simulink library "gnc2_interface_lib"  (R2016b)
settings: Solver=VariableStepAuto  StartTime=0.0  StopTime=10.0  RelTol=1e-3
undefined symbols (not defined in the file): soac_params
libraries: simulink x2, gnc2_lib x1
settings Model: Creator=taylorreynolds  LastModifiedBy=Taylor

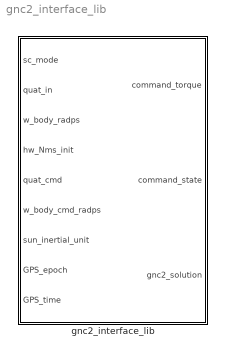
== system gnc2_interface_lib ==
  gnc2_interface_lib : Subsystem

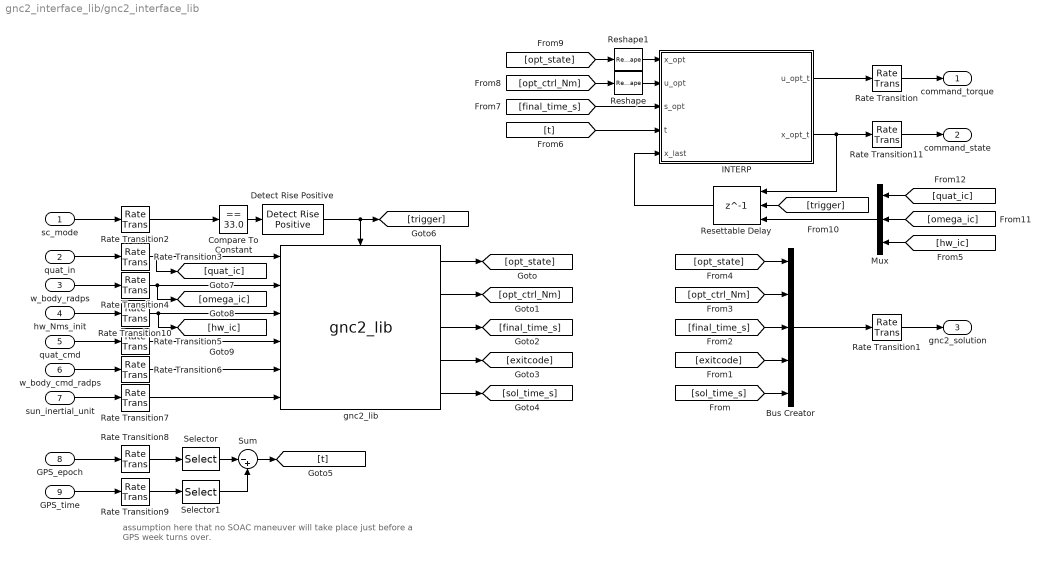
== system gnc2_interface_lib/gnc2_interface_lib ==
  note: assumption here that no SOAC maneuver will take place just
      | before a GPS week turns over.
  sc_mode : Inport
  quat_in : Inport  Port=2
  w_body_radps : Inport  Port=3
  hw_Nms_init : Inport  Port=4
  quat_cmd : Inport  Port=5
  w_body_cmd_radps : Inport  Port=6
  sun_inertial_unit : Inport  Port=7
  GPS_epoch : Inport  Port=8
  GPS_time : Inport  Port=9
  Bus Creator : BusCreator  Inputs=5
  Compare To Constant : simulink/Logic and Bit Operations/Compare To Constant  relop===  const=33.0  OutDataTypeStr=boolean
  Detect Rise Positive : simulink/Logic and Bit Operations/Detect Rise Positive  vinit=0  OutDataTypeStr=boolean
  INTERP : MATLAB Function  TreatAsAtomicUnit=on
  Mux : Mux  Inputs=[4 3 3]
  Rate Transition : RateTransition  X0=soac_params.ic.cmd_torque
  Rate Transition1 : RateTransition
  Rate Transition10 : RateTransition  X0=soac_params.ic.hw_Nms  OutPortSampleTime=soac_params.sample_time_s
  Rate Transition11 : RateTransition  X0=soac_params.ic.cmd_state
  Rate Transition2 : RateTransition  X0=soac_params.ic.sc_mode  OutPortSampleTime=soac_params.sample_time_s
  Rate Transition3 : RateTransition  X0=soac_params.ic.quat_in  OutPortSampleTime=soac_params.sample_time_s
  Rate Transition4 : RateTransition  X0=soac_params.ic.w_body_radps  OutPortSampleTime=soac_params.sample_time_s
  Rate Transition5 : RateTransition  X0=soac_params.ic.quat_cmd  OutPortSampleTime=soac_params.sample_time_s
  Rate Transition6 : RateTransition  X0=soac_params.ic.w_body_cmd_radps  OutPortSampleTime=soac_params.sample_time_s
  Rate Transition7 : RateTransition  X0=soac_params.ic.sun_inertial_unit  OutPortSampleTime=soac_params.sample_time_s
  Rate Transition8 : RateTransition  X0=soac_params.ic.gps_epoch_s  OutPortSampleTime=soac_params.sample_time_s
  Rate Transition9 : RateTransition  X0=soac_params.ic.gps_time_s  OutPortSampleTime=soac_params.sample_time_s
  Resettable Delay : Delay  DelayLength=1  InitialConditionSource=Input port  ExternalReset=Rising
      settings: InputPortMap=u0,r5,p4
  Reshape : Reshape  OutputDimensionality=Customize  OutputDimensions=[3,soac_params.N]
  Reshape1 : Reshape  OutputDimensionality=Customize  OutputDimensions=[10,soac_params.N]
  Selector : Selector  InputPortWidth=2  IndexOptions=Index vector (dialog)  Indices=1  OutputSizes=1
  Selector1 : Selector  InputPortWidth=2  IndexOptions=Index vector (dialog)  Indices=1  OutputSizes=1
  Sum : Sum  Inputs=|-+
  gnc2_lib : gnc2_lib/gnc2_lib
  command_torque : Outport
  command_state : Outport  Port=2
  gnc2_solution : Outport  Port=3
  wires:
  Reshape1/1 -> INTERP/1(x_opt)
  [t] -> INTERP/4(t)
  [final_time_s] -> INTERP/3(s_opt)
  [opt_ctrl_Nm] -> Reshape/1
  [opt_state] -> Reshape1/1
  Reshape/1 -> INTERP/2(u_opt)
  Resettable Delay/1 -> INTERP/5(x_last)
  Rate Transition11/1 -> command_state/1
  INTERP/2(x_opt_t) -> Resettable Delay/1, Rate Transition11/1
  INTERP/1(u_opt_t) -> Rate Transition/1
  quat_in/1 -> Rate Transition3/1
  w_body_radps/1 -> Rate Transition4/1
  quat_cmd/1 -> Rate Transition5/1
  w_body_cmd_radps/1 -> Rate Transition6/1
  sun_inertial_unit/1 -> Rate Transition7/1
  sc_mode/1 -> Rate Transition2/1
  Compare To Constant/1 -> Detect Rise Positive/1
  gnc2_lib/1 -> [opt_state]
  gnc2_lib/5 -> [sol_time_s]
  gnc2_lib/4 -> [exitcode]
  gnc2_lib/3 -> [final_time_s]
  gnc2_lib/2 -> [opt_ctrl_Nm]
  GPS_epoch/1 -> Rate Transition8/1
  GPS_time/1 -> Rate Transition9/1
  Sum/1 -> [t]
  Bus Creator/1 -> Rate Transition1/1
  [sol_time_s] -> Bus Creator/5
  [exitcode] -> Bus Creator/4
  [final_time_s] -> Bus Creator/3
  [opt_ctrl_Nm] -> Bus Creator/2
  [opt_state] -> Bus Creator/1
  Rate Transition/1 -> command_torque/1
  Rate Transition1/1 -> gnc2_solution/1
  Rate Transition2/1 -> Compare To Constant/1
  Rate Transition3/1 -> [quat_ic], gnc2_lib/1
  Rate Transition4/1 -> [omega_ic], gnc2_lib/2
  Rate Transition5/1 -> gnc2_lib/4
  Rate Transition6/1 -> gnc2_lib/5
  Rate Transition7/1 -> gnc2_lib/6
  Rate Transition8/1 -> Selector/1
  Rate Transition9/1 -> Selector1/1
  Selector/1 -> Sum/1
  Selector1/1 -> Sum/2
  Detect Rise Positive/1 -> [trigger], gnc2_lib/Trigger
  Rate Transition10/1 -> [hw_ic], gnc2_lib/3
  hw_Nms_init/1 -> Rate Transition10/1
  [trigger] -> Resettable Delay/2
  [hw_ic] -> Mux/3
  [omega_ic] -> Mux/2
  [quat_ic] -> Mux/1
  Mux/1 -> Resettable Delay/3

== matlab function gnc2_interface_lib/INTERP ==
  data: u_opt_t output size=3; x_opt input; x_opt_t output size=10; u_opt input; s_opt input size=1; t input size=1; x_last input size=10; soac_params parameter
function [u_opt_t,x_opt_t] = soac_INTERP(x_opt,u_opt,s_opt,t,x_last,soac_params)
%#codegen

% parameters
N  = 10;
ut = linspace(0,s_opt,N); % soac_params.N = 10
k  = sum(t>ut); % current interval
J  = [ 0.0338    -4.884e-05 -7.393e-05;
    -4.884e-05  0.0346     7.124e-06;
    -7.393e-05  7.124e-06  0.0075 ]; % kg m2

% Output final state/control if we are beyond the final maneuver time
if ((s_opt>0)&&(t>=s_opt))
    u_opt_t = zeros(3,1);
    x_opt_t = [ x_opt(1:4,N); J\x_opt(5:7,N); x_opt(8:10,N) ];
    return;
end

% Otherwise integrate to current state and interpolate for current control
if ((k>0) && (s_opt>0))
    um      = u_opt(3*(k-1)+(1:3));
    up      = u_opt(3*k+(1:3));
    u       = [reshape(um,3,1) reshape(up,3,1)];
    tspan   = [ ut(k); ut(k+1) ];
    
    % step integrator for x_opt_t
    x_opt_t = rk4_one_step(t,x_last,u,J,tspan,soac_params.sample_time_s);
%     x_opt_t = [ x_opt_t(1:4); J\x_opt_t(5:7); x_opt_t(8:10) ];
%     x_opt_t = [ x_opt(1:4,k); x_opt(5:7,k); x_opt(8:10,k) ];

    % interpolate for control
    u_opt_t = zeros(3,1);
    for i = 1:3
        u_opt_t(i) = interp1(ut,u_opt(i,:),t,'linear');
    end
else
    u_opt_t = zeros(3,1);
    x_opt_t = x_last;
end

end

function x = rk4_one_step(t,x,u,J,tspan,h)

k1 = deriv(t    ,x       ,u,J,tspan);
k2 = deriv(t+h/2,x+h/2*k1,u,J,tspan);
k3 = deriv(t+h/2,x+h/2*k2,u,J,tspan);
k4 = deriv(t+h  ,x+h*k3  ,u,J,tspan);

x = (x+h/6*(k1+2*k2+2*k3+k4));

end

function dx = deriv(t,x,u,J,tspan)

% States
q   = x(1:4)./norm(x(1:4));
q0  = q(1);
qv  = q(2:4);
hb  = x(5:7);
hw  = x(8:10);
w   = J\hb;

% interpolate u_opt at time t
tkm     = tspan(1);
tkp     = tspan(2);
lam_km  = (tkp - t)/(tkp - tkm);
lam_kp  = (t - tkm)/(tkp - tkm);

% Interpolate u
u_tau = lam_km .* u(:,1) + lam_kp .* u(:,2);

% Kinematics & Dynamics
fq  = 0.5 * [ -qv'; skew(qv)+q0*eye(3) ] * w;
fhb = -u_tau + skew(hb+hw) * w;
fhw = u_tau;

dx = [ fq; fhb; fhw ];

end
